simulink model "sampleModel36"  (Simulink 9.1)
settings: Solver=VariableStepAuto  StartTime=0.0  StopTime=10.0  RelTol=1e-3
undefined symbols (not defined in the file): DiscIntNeverNeededParam, Newton, Raphson
libraries: simulink x48
(part 1 of 2)
settings Model: SuppressorTable="22 serialization::archive 11 0 6 0 0 2 8 0 0 0 0 6 0 0 1 0 21 sampleModel36/cfblk78 0 6 0 0 2 8 0 0 0 0 6 41 Simulink:DataType:WarningOverFlowDetected 0 0 0 6 0  0  0 0 0 0 8 20160608 0 0 0 15 23 17 0 1 40 SimulinkFixedPoint:util:Overflowoccurred 0 0 0  0  8 20160608 0 15 23 17 0 1 1 0 21 sampleModel36/cfblk80 2 8 0 41 Simulink:DataType:WarningOverFlowDetected 0 0 0  0  8 20160523 0 10 57 55 0 1 40 SimulinkFixedPoint:util:Overflowoccurred 0 0 0  0  8 20160523 0 10 57 55 0 1"  Creator=DELL  LastModifiedBy=DELL
settings DataIOCC: SaveFormat=Dataset
settings OptimizationCC: LifeSpan=auto
settings DebuggingCC: UnderspecifiedInitializationDetection=Simplified  MergeDetectMultiDrivingBlocksExec=error  SFUnexpectedBacktrackingDiag=error  SFNoUnconditionalDefaultTransitionDiag=error  SFExecutionAtInitializationDiag=warning
settings HardwareCC: ProdBitPerPointer=64  ProdBitPerSizeT=64  ProdBitPerPtrDiffT=64  ProdLargestAtomicFloat=Float  ProdIntDivRoundTo=Zero  ProdEndianess=LittleEndian  ProdWordSize=64  ProdHWDeviceType=Intel->x86-64 (Windows64)
settings ModelReferenceCC: PropagateSignalLabelsOutOfModel=on
settings CodeAppCC: StateflowObjectComments=off
settings GRTTargetCC: TargetLangStandard=C99 (ISO)  CombineOutputUpdateFcns=on  GRTInterface=off
settings ConfigComp: CovMetricSettings=dwe  CovHtmlReporting=off  CovSaveCumulativeToWorkspaceVar=off  CovSaveSingleToWorkspaceVar=off  CovExternalEMLEnable=on

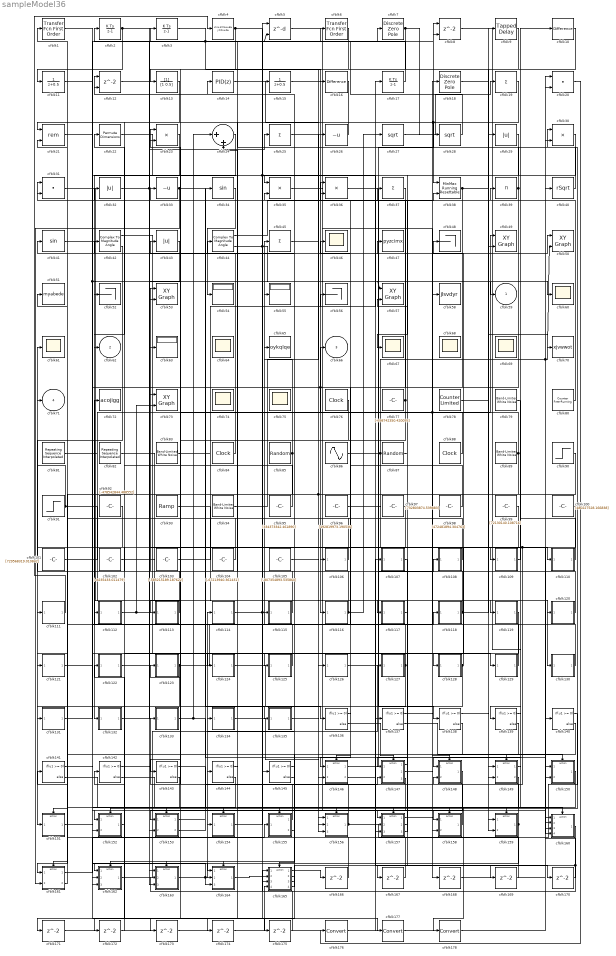
== system sampleModel36 ==
  cfblk1 : simulink/Discrete/Transfer Fcn First Order  PoleZ=0.95  ICPrevOutput=0.0  DoSatur=off
      settings: SourceProductName=Simulink
  cfblk10 : simulink/Discrete/Difference  ICPrevInput=0.0  OutMin=[]  OutMax=[]  OutDataTypeStr=Inherit: Inherit via back propagation  OutDataType=fixdt(1, 16)  OutScaling=2^-10  DoSatur=off
  cfblk100 : Constant  Value=[480227528.166838]  SampleTime=1
  cfblk101 : Constant  Value=[729568319.010842]  SampleTime=1
  cfblk102 : Constant  Value=[-8235433.011479]  SampleTime=1
  cfblk103 : Constant  Value=[-585215189.187622]  SampleTime=1
  cfblk104 : Constant  Value=[-67213940.361431]  SampleTime=1
  cfblk105 : Constant  Value=[-807354893.535860]  SampleTime=1
  cfblk106 : Subsystem
  cfblk107 : Subsystem
  cfblk108 : Subsystem
  cfblk109 : Subsystem
  cfblk11 : DiscreteTransferFcn  SampleTime=1
  cfblk110 : Subsystem
  cfblk111 : Subsystem
  cfblk112 : Subsystem
  cfblk113 : Subsystem
  cfblk114 : Subsystem
  cfblk115 : Subsystem
  cfblk116 : Subsystem
  cfblk117 : Subsystem
  cfblk118 : Subsystem
  cfblk119 : Subsystem
  cfblk12 : Delay  ShowEnablePort=on  SampleTime=1
      settings: InputPortMap=u0,e6
  cfblk120 : Subsystem
  cfblk121 : Subsystem
  cfblk122 : Subsystem
  cfblk123 : Subsystem
  cfblk124 : Subsystem
  cfblk125 : Subsystem
  cfblk126 : Subsystem
  cfblk127 : Subsystem
  cfblk128 : Subsystem
  cfblk129 : Subsystem
  cfblk13 : DiscreteFilter  SampleTime=1
  cfblk130 : Subsystem
  cfblk131 : Subsystem
  cfblk132 : Subsystem
  cfblk133 : Subsystem
  cfblk134 : Subsystem
  cfblk135 : Subsystem
  cfblk{136..145} (10 alike) : If  IfExpression=u1 >= 0  SampleTime=1
  cfblk14 : simulink/Continuous/PID Controller  Controller=PID  TimeDomain=Discrete-time  SampleTime=1  IntegratorMethod=Forward Euler  FilterMethod=Forward Euler  Form=Parallel  UseFilter=on  ControllerParametersSource=internal  P=1  I=1  D=0  N=100  InitialConditionSource=internal  InitialConditionForIntegrator=0  InitialConditionForFilter=0  ExternalReset=none  LimitOutput=off  UpperSaturationLimit=inf  LowerSaturationLimit=-inf  LinearizeAsGain=off  AntiWindupMode=none  Kb=1  TrackingMode=off  Kt=1  PParamMin=[]  PParamMax=[]  IParamMin=[]  IParamMax=[]  DParamMin=[]  DParamMax=[]  NParamMin=[]  NParamMax=[]  KbParamMin=[]  KbParamMax=[]  KtParamMin=[]  KtParamMax=[]  POutMin=[]  POutMax=[]  IOutMin=[]  IOutMax=[]  DOutMin=[]  DOutMax=[]  NOutMin=[]  NOutMax=[]  KbOutMin=[]  KbOutMax=[]  KtOutMin=[]  KtOutMax=[]  IntegratorOutMin=[]  IntegratorOutMax=[]  FilterOutMin=[]  FilterOutMax=[]  SumOutMin=[]  SumOutMax=[]  SumI1OutMin=[]  SumI1OutMax=[]  SumI2OutMin=[]  SumI2OutMax=[]  SumI3OutMin=[]  SumI3OutMax=[]  SumDOutMin=[]  SumDOutMax=[]  SaturationOutMin=[]  SaturationOutMax=[]  IntegratorContinuousStateAttributes=''  IntegratorStateMustResolveToSignalObject=off  IntegratorRTWStateStorageClass=Auto  FilterContinuousStateAttributes=''  FilterStateMustResolveToSignalObject=off  FilterRTWStateStorageClass=Auto  DifferentiatorICPrevScaledInput=0  DifferentiatorOutMin=[]  DifferentiatorOutMax=[]  FilterDiffOutCoefMin=[]  FilterDiffOutCoefMax=[]  SumDenOutMin=[]  SumDenOutMax=[]  SumNumOutMin=[]  SumNumOutMax=[]  ReciprocalOutMin=[]  ReciprocalOutMax=[]  DivideOutMin=[]  DivideOutMax=[]  TunerSelectOption=Transfer Function Based (PID Tuner App)
  cfblk146 : Subsystem  TreatAsAtomicUnit=on
  cfblk147 : Subsystem  TreatAsAtomicUnit=on
  cfblk148 : Subsystem  TreatAsAtomicUnit=on
  cfblk149 : Subsystem  TreatAsAtomicUnit=on
  cfblk15 : DiscreteTransferFcn  SampleTime=1
  cfblk150 : Subsystem  TreatAsAtomicUnit=on
  cfblk151 : Subsystem  TreatAsAtomicUnit=on
  cfblk152 : Subsystem  TreatAsAtomicUnit=on
  cfblk153 : Subsystem  TreatAsAtomicUnit=on
  cfblk154 : Subsystem  TreatAsAtomicUnit=on
  cfblk155 : Subsystem  TreatAsAtomicUnit=on
  cfblk156 : Subsystem  TreatAsAtomicUnit=on
  cfblk157 : Subsystem  TreatAsAtomicUnit=on
  cfblk158 : Subsystem  TreatAsAtomicUnit=on
  cfblk159 : Subsystem  TreatAsAtomicUnit=on
  cfblk16 : simulink/Discrete/Difference  ICPrevInput=0.0  OutMin=[]  OutMax=[]  OutDataTypeStr=Inherit: Inherit via back propagation  OutDataType=fixdt(1, 16)  OutScaling=2^-10  DoSatur=off
  cfblk160 : Subsystem  TreatAsAtomicUnit=on
  cfblk161 : Subsystem  TreatAsAtomicUnit=on
  cfblk162 : Subsystem  TreatAsAtomicUnit=on
  cfblk163 : Subsystem  TreatAsAtomicUnit=on
  cfblk164 : Subsystem  TreatAsAtomicUnit=on
  cfblk165 : Subsystem  TreatAsAtomicUnit=on
  cfblk{166..175} (10 alike) : Delay  SampleTime=1
  cfblk17 : DiscreteIntegrator  ICPrevOutput=DiscIntNeverNeededParam  ICPrevScaledInput=DiscIntNeverNeededParam
  cfblk176 : DataTypeConversion
  cfblk177 : DataTypeConversion
  cfblk178 : DataTypeConversion
  cfblk18 : DiscreteZeroPole  Poles=[0 0.5]  Gain=1
  cfblk{19,25,37,45} (4 alike) : Sum  Inputs=+
  cfblk2 : DiscreteIntegrator  ICPrevOutput=DiscIntNeverNeededParam  ICPrevScaledInput=DiscIntNeverNeededParam
  cfblk20 : DotProduct  InputSameDT=on  OutDataTypeStr=Inherit: Inherit via internal rule
  cfblk21 : Math  Operator=rem  SaturateOnIntegerOverflow=on
  cfblk22 : PermuteDimensions
  cfblk23 : Product  Inputs=**
  cfblk24 : Sum  Inputs=|++
  cfblk26 : UnaryMinus
  cfblk27 : Sqrt  SaturateOnIntegerOverflow=on
  cfblk28 : Sqrt  SaturateOnIntegerOverflow=on
  cfblk29 : Abs
  cfblk3 : DiscreteIntegrator  ICPrevOutput=DiscIntNeverNeededParam  ICPrevScaledInput=DiscIntNeverNeededParam
  cfblk30 : Product
  cfblk31 : DotProduct  InputSameDT=on  OutDataTypeStr=Inherit: Inherit via internal rule
  cfblk32 : Abs
  cfblk33 : UnaryMinus
  cfblk34 : Trigonometry
  cfblk35 : Product
  cfblk36 : Product
  cfblk38 : simulink/Math Operations/MinMax Running Resettable  Function=min  vinit=0.0
  cfblk39 : Product  Inputs=*
  cfblk4 : DiscreteStateSpace
  cfblk40 : Sqrt  Operator=rSqrt  AlgorithmType=Newton-Raphson  SaturateOnIntegerOverflow=on
  cfblk41 : Trigonometry
  cfblk42 : ComplexToMagnitudeAngle
  cfblk43 : Abs
  cfblk44 : ComplexToMagnitudeAngle
  cfblk{46,60..61,64,67..69,74..75} (9 alike) : Scope
      cfblk64 settings: Floating=on
      cfblk68 settings: Floating=on
      cfblk69 settings: Floating=on
      cfblk74 settings: Floating=on
      cfblk75 settings: Floating=on
  cfblk47 : ToWorkspace  VariableName=pyzcimx  SaveFormat=Timeseries  SampleTime=-1
  cfblk48 : Terminator
  cfblk{49..50,53,57,73} (5 alike) : simulink/Sinks/XY Graph  xmin=-1  xmax=1  ymin=-1  ymax=1  st=-1
  cfblk5 : Delay  DelayLengthSource=Input port  SampleTime=1
      settings: InputPortMap=u0,p1
  cfblk51 : ToWorkspace  VariableName=myabede  SaveFormat=Timeseries  SampleTime=-1
  cfblk52 : Terminator
  cfblk54 : Display
  cfblk55 : Display
  cfblk56 : Terminator
  cfblk58 : ToWorkspace  VariableName=jlsvdyr  SaveFormat=Timeseries  SampleTime=-1
  cfblk6 : simulink/Discrete/Transfer Fcn First Order  PoleZ=0.95  ICPrevOutput=0.0  DoSatur=off
      settings: SourceProductName=Simulink
  cfblk63 : Display
  cfblk65 : ToWorkspace  VariableName=oykqlqe  SaveFormat=Timeseries  SampleTime=-1
  cfblk7 : DiscreteZeroPole  Poles=[0 0.5]  Gain=1
  cfblk70 : ToWorkspace  VariableName=xjvwwot  SaveFormat=Timeseries  SampleTime=-1
  cfblk72 : ToWorkspace  VariableName=acojigg  SaveFormat=Timeseries  SampleTime=-1
  cfblk76 : DigitalClock
  cfblk77 : Constant  Value=[-698742350.420095]  SampleTime=1
  cfblk78 : simulink/Sources/Counter Limited  uplimit=[563.000000]  tsamp=-1
  cfblk79 : simulink/Sources/Band-Limited White Noise  Cov=[5262245646.947961]  Ts=0.1  seed=[7499573642.000000]
  cfblk8 : Delay  ShowEnablePort=on  SampleTime=1
      settings: InputPortMap=u0,e6
  cfblk80 : simulink/Sources/Counter Free-Running  NumBits=[10.000000]  tsamp=-1
  cfblk81 : simulink/Sources/Repeating Sequence Interpolated  OutValues=[-717569786.337497, -786951545.619581, 871859825.205165, -978024908.591797, -592437085.964163]  TimeValues=[0 0.1 0.5 0.6 1].'  LookUpMeth=Use Input Below  tsamp=0.01  OutMin=[]  OutMax=[]  OutDataTypeStr=double  OutputDataTypeScalingMode=double  OutDataType=fixdt(0,8)  OutScaling=2^-10
  cfblk82 : simulink/Sources/Repeating Sequence Interpolated  OutValues=[-154038240.023456, 915570522.285018, -432332103.291962, 774629816.872916, -868714883.246416]  TimeValues=[0 0.1 0.5 0.6 1].'  LookUpMeth=Use Input Above  tsamp=0.01  OutMin=[]  OutMax=[]  OutDataTypeStr=double  OutputDataTypeScalingMode=double  OutDataType=fixdt(0,8)  OutScaling=2^-10
  cfblk83 : simulink/Sources/Band-Limited White Noise  Cov=[2765316876.474610]  Ts=0.1  seed=[5715553858.000000]
  cfblk84 : DigitalClock
  cfblk85 : UniformRandomNumber  Minimum=[-3503548894.777228]  Maximum=[8747219414.346481]  Seed=[48755141.000000]  SampleTime=0.1
  cfblk86 : Sin  Amplitude=[-627808321.925341]  Bias=[-301483454.666432]  SampleTime=0
  cfblk87 : UniformRandomNumber  Minimum=[-5653446870.603408]  Maximum=[6046751050.321515]  Seed=[57719394.000000]  SampleTime=0.1
  cfblk88 : DigitalClock
  cfblk89 : simulink/Sources/Band-Limited White Noise  Cov=[5063504057.072619]  Ts=0.1  seed=[2488343886.000000]
  cfblk9 : simulink/Discrete/Tapped Delay  vinit=0.0  samptime=-1  NumDelays=1  DelayOrder=Oldest  includeCurrent=off
  cfblk90 : Step  Time=[27.000000]  Before=[545712773.558107]  After=[102090399.807930]  SampleTime=0
  cfblk91 : Step  Time=[37.000000]  Before=[895402550.988094]  After=[591374171.611668]  SampleTime=0
  cfblk92 : Constant  Value=[-478542844.488552]  SampleTime=1
  cfblk93 : simulink/Sources/Ramp  slope=[-3591.772150]  start=[40.612428]  InitialOutput=[471167.394474]
  cfblk94 : simulink/Sources/Band-Limited White Noise  Cov=[7229783405.351925]  Ts=0.1  seed=[743836585.000000]
  cfblk95 : Constant  Value=[334373342.461890]  SampleTime=1
  cfblk96 : Constant  Value=[492819973.190536]  SampleTime=1
  cfblk97 : Constant  Value=[732803874.539883]  SampleTime=1
  cfblk98 : Constant  Value=[472481894.304763]  SampleTime=1
  cfblk99 : Constant  Value=[72130140.108716]  SampleTime=1
  cfblk59 : Outport
  cfblk62 : Outport  Port=2
  cfblk66 : Outport  Port=3
  cfblk71 : Outport  Port=4
  wires:
  cfblk42/1 -> cfblk129/1(cfblk1)
  cfblk23/1 -> cfblk132/1(cfblk1)
  cfblk16/1 -> cfblk33/1
  cfblk106/1(cfblk2) -> cfblk53/1
  cfblk8/1 -> cfblk148/1(cfblk1)
  cfblk100/1 -> cfblk133/1(cfblk1), cfblk128/1(cfblk1)
  cfblk91/1 -> cfblk61/1, cfblk160/3(cfblk14)
  cfblk116/1(cfblk2) -> cfblk27/1, cfblk24/2
  cfblk163/1(cfblk2) -> cfblk114/1(cfblk1)
  cfblk109/1(cfblk2) -> cfblk10/1
  cfblk36/1 -> cfblk138/1
  cfblk17/1 -> cfblk2/1
  cfblk126/1(cfblk2) -> cfblk8/1
  cfblk5/1 -> cfblk158/1(cfblk1)
  cfblk27/1 -> cfblk19/1
  cfblk78/1 -> cfblk149/1(cfblk1)
  cfblk146/1(cfblk2) -> cfblk108/1(cfblk1)
  cfblk7/1 -> cfblk113/1(cfblk1), cfblk28/1
  cfblk124/1(cfblk2) -> cfblk136/1
  cfblk6/1 -> cfblk116/1(cfblk1)
  cfblk81/1 -> cfblk49/1
  cfblk32/1 -> cfblk110/1(cfblk1), cfblk8/2
  cfblk31/1 -> cfblk119/1(cfblk1)
  cfblk118/1(cfblk2) -> cfblk9/1, cfblk73/1
  cfblk158/1(cfblk2) -> cfblk123/1(cfblk1)
  cfblk120/1(cfblk2) -> cfblk71/1
  cfblk25/1 -> cfblk59/1
  cfblk132/1(cfblk2) -> cfblk47/1
  cfblk130/1(cfblk2) -> cfblk31/1
  cfblk39/1 -> cfblk12/1, cfblk163/3(cfblk17)
  cfblk83/1 -> cfblk17/1
  cfblk37/1 -> cfblk146/1(cfblk1)
  cfblk4/1 -> cfblk13/1, cfblk109/1(cfblk1)
  cfblk122/1(cfblk2) -> cfblk50/1
  cfblk135/1(cfblk2) -> cfblk149/2(cfblk11)
  cfblk111/1(cfblk2) -> cfblk4/1
  cfblk96/1 -> cfblk159/1(cfblk1)
  cfblk112/1(cfblk2) -> cfblk25/1, cfblk73/2
  cfblk162/1(cfblk2) -> cfblk127/1(cfblk1)
  cfblk85/1 -> cfblk143/1, cfblk65/1
  cfblk79/1 -> cfblk139/1
  cfblk99/1 -> cfblk162/1(cfblk1)
  cfblk129/1(cfblk2) -> cfblk45/1
  cfblk77/1 -> cfblk164/1(cfblk1), cfblk32/1
  cfblk12/1 -> cfblk163/1(cfblk1)
  cfblk24/1 -> cfblk52/1
  cfblk13/1 -> cfblk62/1
  cfblk103/1 -> cfblk5/1
  cfblk34/1 -> cfblk54/1
  cfblk2/1 -> cfblk11/1, cfblk160/4(cfblk15)
  cfblk87/1 -> cfblk37/1
  cfblk155/1(cfblk2) -> cfblk43/1
  cfblk115/1(cfblk2) -> cfblk55/1
  cfblk15/1 -> cfblk130/1(cfblk1)
  cfblk127/1(cfblk2) -> cfblk46/1, cfblk173/1
  cfblk108/1(cfblk2) -> cfblk63/1
  cfblk101/1 -> cfblk29/1, cfblk18/1
  cfblk43/1 -> cfblk53/2
  cfblk10/1 -> cfblk49/2
  cfblk3/1 -> cfblk16/1, cfblk5/2
  cfblk128/1(cfblk2) -> cfblk48/1, cfblk157/1(cfblk1)
  cfblk41/1 -> cfblk137/1
  cfblk97/1 -> cfblk151/1(cfblk1)
  cfblk29/1 -> cfblk67/1
  cfblk95/1 -> cfblk22/1
  cfblk110/1(cfblk2) -> cfblk39/1
  cfblk160/1(cfblk2) -> cfblk163/2(cfblk16), cfblk171/1
  cfblk94/1 -> cfblk26/1
  cfblk134/1(cfblk2) -> cfblk146/2(cfblk13)
  cfblk131/1(cfblk2) -> cfblk7/1
  cfblk28/1 -> cfblk6/1
  cfblk42/2 -> cfblk111/1(cfblk1)
  cfblk92/1 -> cfblk121/1(cfblk1)
  cfblk89/1 -> cfblk131/1(cfblk1), cfblk23/2
  cfblk156/1(cfblk2) -> cfblk30/1, cfblk23/1
  cfblk18/1 -> cfblk120/1(cfblk1)
  cfblk21/1 -> cfblk164/2(cfblk8), cfblk164/3(cfblk9), cfblk57/1
  cfblk26/1 -> cfblk21/1
  cfblk35/1 -> cfblk158/2(cfblk14)
  cfblk98/1 -> cfblk36/1
  cfblk82/1 -> cfblk150/1(cfblk1)
  cfblk107/1(cfblk2) -> cfblk147/1(cfblk1)
  cfblk161/1(cfblk2) -> cfblk155/1(cfblk1)
  cfblk113/1(cfblk2) -> cfblk42/1
  cfblk14/1 -> cfblk156/1(cfblk1)
  cfblk165/2(cfblk11) -> cfblk12/2
  cfblk152/1(cfblk2) -> cfblk122/1(cfblk1)
  cfblk104/1 -> cfblk41/1
  cfblk154/1(cfblk2) -> cfblk56/1
  cfblk161/2(cfblk10) -> cfblk51/1
  cfblk117/1(cfblk2) -> cfblk57/2
  cfblk44/1 -> cfblk36/2
  cfblk93/1 -> cfblk159/2(cfblk17)
  cfblk121/1(cfblk2) -> cfblk118/1(cfblk1)
  cfblk90/1 -> cfblk156/2(cfblk11), cfblk153/2(cfblk13)
  cfblk159/1(cfblk2) -> cfblk144/1, cfblk162/2(cfblk8)
  cfblk165/3(cfblk12) -> cfblk134/1(cfblk1)
  cfblk102/1 -> cfblk126/1(cfblk1)
  cfblk149/1(cfblk2) -> cfblk148/2(cfblk10)
  cfblk19/1 -> cfblk38/1, cfblk124/1(cfblk1)
  cfblk38/1 -> cfblk106/1(cfblk1), cfblk162/3(cfblk9), cfblk70/1
  cfblk1/1 -> cfblk35/1
  cfblk40/1 -> cfblk3/1
  cfblk133/1(cfblk2) -> cfblk150/2(cfblk13), cfblk24/1
  cfblk44/2 -> cfblk15/1, cfblk60/1
  cfblk125/1(cfblk2) -> cfblk72/1
  cfblk80/1 -> cfblk1/1
  cfblk153/1(cfblk2) -> cfblk34/1
  cfblk105/1 -> cfblk117/1(cfblk1)
  cfblk123/1(cfblk2) -> cfblk58/1, cfblk161/1(cfblk1)
  cfblk84/1 -> cfblk21/2
  cfblk45/1 -> cfblk38/2
  cfblk165/4(cfblk13) -> cfblk44/1
  cfblk157/2(cfblk14) -> cfblk112/1(cfblk1)
  cfblk86/1 -> cfblk50/2, cfblk40/1, cfblk160/2(cfblk13)
  cfblk76/1 -> cfblk153/1(cfblk1)
  cfblk22/1 -> cfblk115/1(cfblk1), cfblk145/1, cfblk157/2(cfblk12)
  cfblk11/1 -> cfblk125/1(cfblk1)
  cfblk157/3(cfblk15) -> cfblk31/2
  cfblk9/1 -> cfblk156/3(cfblk12)
  cfblk164/1(cfblk2) -> cfblk165/2(cfblk8)
  cfblk30/1 -> cfblk165/3(cfblk9)
  cfblk88/1 -> cfblk66/1
  cfblk33/1 -> cfblk135/1(cfblk1), cfblk161/2(cfblk9)
  cfblk155/2(cfblk13) -> cfblk14/1
  cfblk153/2(cfblk14) -> cfblk147/2(cfblk14)
  cfblk148/1(cfblk2) -> cfblk152/1(cfblk1)
  cfblk147/3(cfblk16) -> cfblk152/2(cfblk8)
  cfblk136/1 -> cfblk146/Action
  cfblk136/2 -> cfblk147/Action
  cfblk137/1 -> cfblk148/Action
  cfblk137/2 -> cfblk149/Action
  cfblk138/1 -> cfblk150/Action
  cfblk138/2 -> cfblk151/Action
  cfblk139/1 -> cfblk152/Action
  cfblk139/2 -> cfblk153/Action
  cfblk140/1 -> cfblk154/Action
  cfblk140/2 -> cfblk155/Action
  cfblk141/1 -> cfblk156/Action
  cfblk141/2 -> cfblk157/Action
  cfblk142/1 -> cfblk158/Action
  cfblk142/2 -> cfblk159/Action
  cfblk143/1 -> cfblk160/Action
  cfblk143/2 -> cfblk161/Action
  cfblk144/1 -> cfblk162/Action
  cfblk144/2 -> cfblk163/Action
  cfblk145/1 -> cfblk164/Action
  cfblk145/2 -> cfblk165/Action
  cfblk165/1(cfblk2) -> cfblk166/1
  cfblk166/1 -> cfblk154/1(cfblk1)
  cfblk147/1(cfblk2) -> cfblk167/1
  cfblk167/1 -> cfblk35/2
  cfblk147/2(cfblk15) -> cfblk168/1
  cfblk168/1 -> cfblk30/2
  cfblk146/2(cfblk14) -> cfblk169/1
  cfblk169/1 -> cfblk141/1
  cfblk157/1(cfblk2) -> cfblk170/1
  cfblk170/1 -> cfblk160/1(cfblk1)
  cfblk171/1 -> cfblk157/3(cfblk13)
  cfblk119/1(cfblk2) -> cfblk172/1
  cfblk172/1 -> cfblk142/1
  cfblk173/1 -> cfblk165/4(cfblk10)
  cfblk150/1(cfblk2) -> cfblk174/1
  cfblk174/1 -> cfblk140/1
  cfblk151/1(cfblk2) -> cfblk175/1
  cfblk175/1 -> cfblk165/1(cfblk1)
  cfblk20/1 -> cfblk176/1
  cfblk176/1 -> cfblk107/1(cfblk1)
  cfblk114/1(cfblk2) -> cfblk177/1
  cfblk177/1 -> cfblk20/1
  cfblk149/2(cfblk12) -> cfblk178/1
  cfblk178/1 -> cfblk20/2

== system sampleModel36/cfblk106 ==
  cfblk1 : Inport
  cfblk2 : Outport
  wires:
  cfblk1/1 -> cfblk2/1

== system sampleModel36/cfblk107 ==
  cfblk1 : Inport
  cfblk2 : Outport
  wires:
  cfblk1/1 -> cfblk2/1

== system sampleModel36/cfblk108 ==
  cfblk1 : Inport
  cfblk2 : Outport
  wires:
  cfblk1/1 -> cfblk2/1

== system sampleModel36/cfblk109 ==
  cfblk1 : Inport
  cfblk2 : Outport
  wires:
  cfblk1/1 -> cfblk2/1

== system sampleModel36/cfblk110 ==
  cfblk1 : Inport
  cfblk2 : Outport
  wires:
  cfblk1/1 -> cfblk2/1

== system sampleModel36/cfblk111 ==
  cfblk1 : Inport
  cfblk2 : Outport
  wires:
  cfblk1/1 -> cfblk2/1

== system sampleModel36/cfblk112 ==
  cfblk1 : Inport
  cfblk2 : Outport
  wires:
  cfblk1/1 -> cfblk2/1

== system sampleModel36/cfblk113 ==
  cfblk1 : Inport
  cfblk2 : Outport
  wires:
  cfblk1/1 -> cfblk2/1

== system sampleModel36/cfblk114 ==
  cfblk1 : Inport
  cfblk2 : Outport
  wires:
  cfblk1/1 -> cfblk2/1

== system sampleModel36/cfblk115 ==
  cfblk1 : Inport
  cfblk2 : Outport
  wires:
  cfblk1/1 -> cfblk2/1

== system sampleModel36/cfblk116 ==
  cfblk1 : Inport
  cfblk2 : Outport
  wires:
  cfblk1/1 -> cfblk2/1

== system sampleModel36/cfblk117 ==
  cfblk1 : Inport
  cfblk2 : Outport
  wires:
  cfblk1/1 -> cfblk2/1

== system sampleModel36/cfblk118 ==
  cfblk1 : Inport
  cfblk2 : Outport
  wires:
  cfblk1/1 -> cfblk2/1

== system sampleModel36/cfblk119 ==
  cfblk1 : Inport
  cfblk2 : Outport
  wires:
  cfblk1/1 -> cfblk2/1

== system sampleModel36/cfblk120 ==
  cfblk1 : Inport
  cfblk2 : Outport
  wires:
  cfblk1/1 -> cfblk2/1

== system sampleModel36/cfblk121 ==
  cfblk1 : Inport
  cfblk2 : Outport
  wires:
  cfblk1/1 -> cfblk2/1

== system sampleModel36/cfblk122 ==
  cfblk1 : Inport
  cfblk2 : Outport
  wires:
  cfblk1/1 -> cfblk2/1

== system sampleModel36/cfblk123 ==
  cfblk1 : Inport
  cfblk2 : Outport
  wires:
  cfblk1/1 -> cfblk2/1

== system sampleModel36/cfblk124 ==
  cfblk1 : Inport
  cfblk2 : Outport
  wires:
  cfblk1/1 -> cfblk2/1

== system sampleModel36/cfblk125 ==
  cfblk1 : Inport
  cfblk2 : Outport
  wires:
  cfblk1/1 -> cfblk2/1

== system sampleModel36/cfblk126 ==
  cfblk1 : Inport
  cfblk2 : Outport
  wires:
  cfblk1/1 -> cfblk2/1

== system sampleModel36/cfblk127 ==
  cfblk1 : Inport
  cfblk2 : Outport
  wires:
  cfblk1/1 -> cfblk2/1

== system sampleModel36/cfblk128 ==
  cfblk1 : Inport
  cfblk2 : Outport
  wires:
  cfblk1/1 -> cfblk2/1

== system sampleModel36/cfblk129 ==
  cfblk1 : Inport
  cfblk2 : Outport
  wires:
  cfblk1/1 -> cfblk2/1

== system sampleModel36/cfblk130 ==
  cfblk1 : Inport
  cfblk2 : Outport
  wires:
  cfblk1/1 -> cfblk2/1

== system sampleModel36/cfblk131 ==
  cfblk1 : Inport
  cfblk2 : Outport
  wires:
  cfblk1/1 -> cfblk2/1

== system sampleModel36/cfblk132 ==
  cfblk1 : Inport
  cfblk2 : Outport
  wires:
  cfblk1/1 -> cfblk2/1

== system sampleModel36/cfblk133 ==
  cfblk1 : Inport
  cfblk2 : Outport
  wires:
  cfblk1/1 -> cfblk2/1

== system sampleModel36/cfblk134 ==
  cfblk1 : Inport
  cfblk2 : Outport
  wires:
  cfblk1/1 -> cfblk2/1

== system sampleModel36/cfblk135 ==
  cfblk1 : Inport
  cfblk2 : Outport
  wires:
  cfblk1/1 -> cfblk2/1

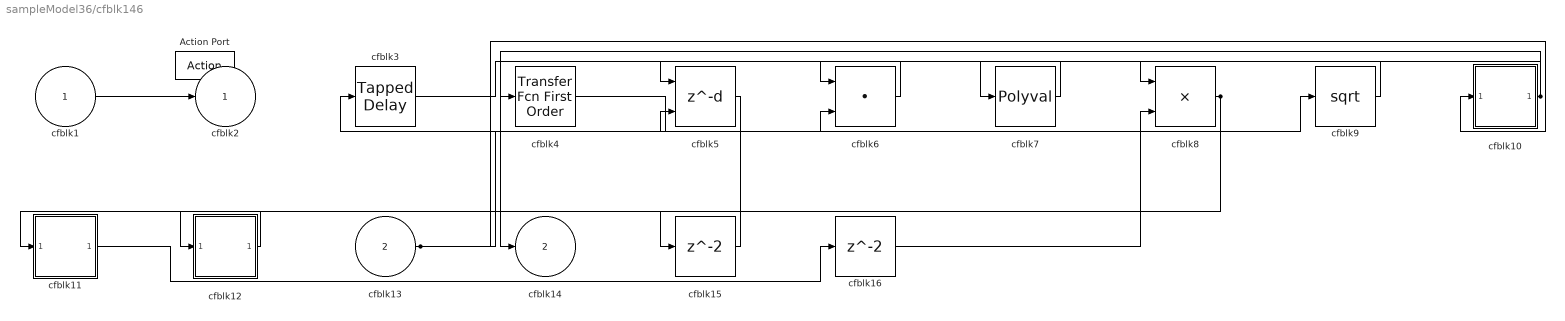
== system sampleModel36/cfblk146 ==
  cfblk1 : Inport
  cfblk13 : Inport  Port=2
  Action Port : ActionPort  ActionType=then
  cfblk10 : Subsystem
  cfblk11 : Subsystem
  cfblk12 : Subsystem
  cfblk15 : Delay
  cfblk16 : Delay
  cfblk3 : simulink/Discrete/Tapped Delay  vinit=0.0  samptime=-1  NumDelays=1  DelayOrder=Oldest  includeCurrent=off
  cfblk4 : simulink/Discrete/Transfer Fcn First Order  PoleZ=0.95  ICPrevOutput=0.0  DoSatur=off
      settings: SourceProductName=Simulink
  cfblk5 : Delay  DelayLengthSource=Input port
      settings: InputPortMap=u0,p1
  cfblk6 : DotProduct  InputSameDT=on  OutDataTypeStr=Inherit: Inherit via internal rule
  cfblk7 : Polyval  Coefs=[ +2.081618890e-019, -1.441693666e-014, +4.719686976e-010, -8.536869453e-006, +1.621573104e-001, -8.087801117e+001 ]
  cfblk8 : Product  Inputs=**
  cfblk9 : Sqrt  SaturateOnIntegerOverflow=on
  cfblk2 : Outport
  cfblk14 : Outport  Port=2
  wires:
  cfblk12/1(cfblk2) -> cfblk11/1(cfblk1)
  cfblk9/1 -> cfblk8/1
  cfblk10/1(cfblk2) -> cfblk14/1, cfblk7/1
  cfblk13/1 -> cfblk10/1(cfblk1), cfblk5/2
  cfblk6/1 -> cfblk5/1
  cfblk7/1 -> cfblk4/1
  cfblk4/1 -> cfblk9/1
  cfblk1/1 -> cfblk2/1
  cfblk3/1 -> cfblk6/1
  cfblk8/1 -> cfblk12/1(cfblk1), cfblk6/2
  cfblk5/1 -> cfblk15/1
  cfblk15/1 -> cfblk3/1
  cfblk11/1(cfblk2) -> cfblk16/1
  cfblk16/1 -> cfblk8/2

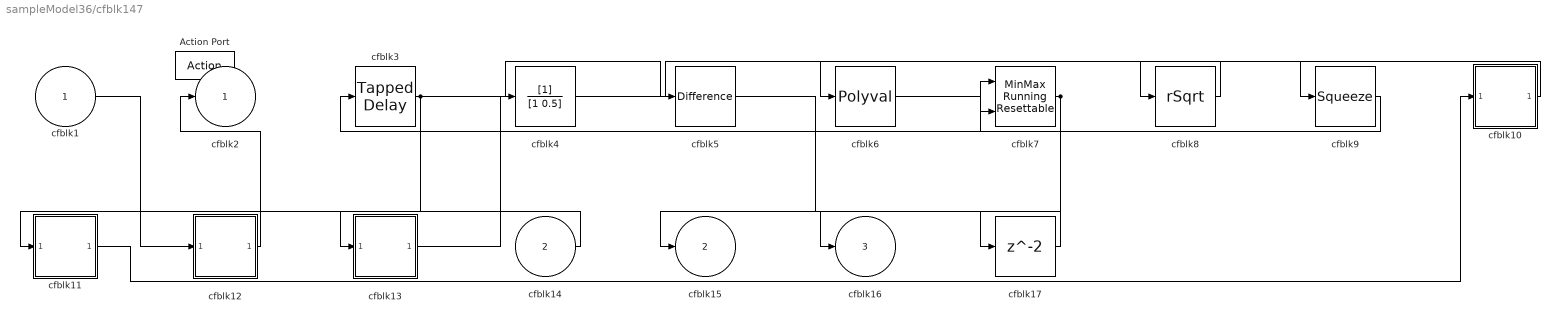
== system sampleModel36/cfblk147 ==
  cfblk1 : Inport
  cfblk14 : Inport  Port=2
  Action Port : ActionPort  ActionType=else
  cfblk10 : Subsystem
  cfblk11 : Subsystem
  cfblk12 : Subsystem
  cfblk13 : Subsystem
  cfblk17 : Delay
  cfblk3 : simulink/Discrete/Tapped Delay  vinit=0.0  samptime=-1  NumDelays=1  DelayOrder=Oldest  includeCurrent=off
  cfblk4 : DiscreteFilter
  cfblk5 : simulink/Discrete/Difference  ICPrevInput=0.0  OutMin=[]  OutMax=[]  OutDataTypeStr=Inherit: Inherit via back propagation  OutDataType=fixdt(1, 16)  OutScaling=2^-10  DoSatur=off
  cfblk6 : Polyval  Coefs=[ +2.081618890e-019, -1.441693666e-014, +4.719686976e-010, -8.536869453e-006, +1.621573104e-001, -8.087801117e+001 ]
  cfblk7 : simulink/Math Operations/MinMax Running Resettable  Function=min  vinit=0.0
  cfblk8 : Sqrt  Operator=rSqrt  AlgorithmType=Newton-Raphson  SaturateOnIntegerOverflow=on
  cfblk9 : Squeeze
  cfblk2 : Outport
  cfblk15 : Outport  Port=2
  cfblk16 : Outport  Port=3
  wires:
  cfblk4/1 -> cfblk9/1
  cfblk9/1 -> cfblk7/1
  cfblk8/1 -> cfblk6/1
  cfblk12/1(cfblk2) -> cfblk2/1
  cfblk3/1 -> cfblk5/1, cfblk11/1(cfblk1)
  cfblk10/1(cfblk2) -> cfblk8/1
  cfblk6/1 -> cfblk7/2
  cfblk1/1 -> cfblk12/1(cfblk1)
  cfblk14/1 -> cfblk13/1(cfblk1)
  cfblk7/1 -> cfblk16/1, cfblk15/1
  cfblk13/1(cfblk2) -> cfblk4/1
  cfblk11/1(cfblk2) -> cfblk10/1(cfblk1)
  cfblk5/1 -> cfblk17/1
  cfblk17/1 -> cfblk3/1

== system sampleModel36/cfblk148 ==
  cfblk1 : Inport
  cfblk10 : Inport  Port=2
  Action Port : ActionPort  ActionType=then
  cfblk3 : Product  Inputs=**
  cfblk4 : DotProduct  InputSameDT=on  OutDataTypeStr=Inherit: Inherit via internal rule
  cfblk5 : Product
  cfblk6 : Sqrt  SaturateOnIntegerOverflow=on
  cfblk7 : Constant  Value=[530901594.292365]  SampleTime=1
  cfblk8 : Subsystem
  cfblk9 : Subsystem
  cfblk2 : Outport
  wires:
  cfblk5/1 -> cfblk8/1(cfblk1)
  cfblk10/1 -> cfblk9/1(cfblk1)
  cfblk8/1(cfblk2) -> cfblk4/1
  cfblk3/1 -> cfblk6/1
  cfblk6/1 -> cfblk4/2
  cfblk7/1 -> cfblk5/1, cfblk5/2
  cfblk4/1 -> cfblk2/1
  cfblk9/1(cfblk2) -> cfblk3/1
  cfblk1/1 -> cfblk3/2

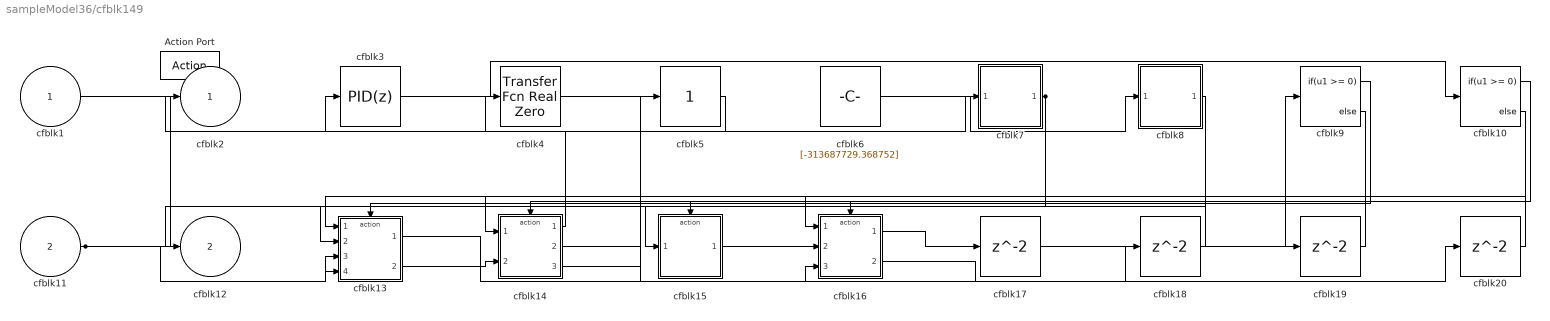
== system sampleModel36/cfblk149 ==
  cfblk1 : Inport
  cfblk11 : Inport  Port=2
  Action Port : ActionPort  ActionType=else
  cfblk10 : If  IfExpression=u1 >= 0  SampleTime=1
  cfblk13 : Subsystem  TreatAsAtomicUnit=on
  cfblk14 : Subsystem  TreatAsAtomicUnit=on
  cfblk15 : Subsystem  TreatAsAtomicUnit=on
  cfblk16 : Subsystem  TreatAsAtomicUnit=on
  cfblk{17..20} (4 alike) : Delay
  cfblk3 : simulink/Continuous/PID Controller  Controller=PID  TimeDomain=Discrete-time  SampleTime=-1  IntegratorMethod=Forward Euler  FilterMethod=Forward Euler  Form=Parallel  UseFilter=on  ControllerParametersSource=internal  P=1  I=1  D=0  N=100  InitialConditionSource=internal  InitialConditionForIntegrator=0  InitialConditionForFilter=0  ExternalReset=none  LimitOutput=off  UpperSaturationLimit=inf  LowerSaturationLimit=-inf  LinearizeAsGain=off  AntiWindupMode=none  Kb=1  TrackingMode=off  Kt=1  PParamMin=[]  PParamMax=[]  IParamMin=[]  IParamMax=[]  DParamMin=[]  DParamMax=[]  NParamMin=[]  NParamMax=[]  KbParamMin=[]  KbParamMax=[]  KtParamMin=[]  KtParamMax=[]  POutMin=[]  POutMax=[]  IOutMin=[]  IOutMax=[]  DOutMin=[]  DOutMax=[]  NOutMin=[]  NOutMax=[]  KbOutMin=[]  KbOutMax=[]  KtOutMin=[]  KtOutMax=[]  IntegratorOutMin=[]  IntegratorOutMax=[]  FilterOutMin=[]  FilterOutMax=[]  SumOutMin=[]  SumOutMax=[]  SumI1OutMin=[]  SumI1OutMax=[]  SumI2OutMin=[]  SumI2OutMax=[]  SumI3OutMin=[]  SumI3OutMax=[]  SumDOutMin=[]  SumDOutMax=[]  SaturationOutMin=[]  SaturationOutMax=[]  IntegratorContinuousStateAttributes=''  IntegratorStateMustResolveToSignalObject=off  IntegratorRTWStateStorageClass=Auto  FilterContinuousStateAttributes=''  FilterStateMustResolveToSignalObject=off  FilterRTWStateStorageClass=Auto  DifferentiatorICPrevScaledInput=0  DifferentiatorOutMin=[]  DifferentiatorOutMax=[]  FilterDiffOutCoefMin=[]  FilterDiffOutCoefMax=[]  SumDenOutMin=[]  SumDenOutMax=[]  SumNumOutMin=[]  SumNumOutMax=[]  ReciprocalOutMin=[]  ReciprocalOutMax=[]  DivideOutMin=[]  DivideOutMax=[]  TunerSelectOption=Transfer Function Based (PID Tuner App)
  cfblk4 : simulink/Discrete/Transfer Fcn Real Zero  ZeroZ=0.75  ICPrevInput=0.0  DoSatur=off
      settings: SourceProductName=Simulink  SourceProductBaseCode=SL
  cfblk5 : simulink/Math Operations/Slider Gain  gain=1  low=0  high=2
  cfblk6 : Constant  Value=[-313687729.368752]  SampleTime=1
  cfblk7 : Subsystem
  cfblk8 : Subsystem
  cfblk9 : If  IfExpression=u1 >= 0  SampleTime=1
  cfblk2 : Outport
  cfblk12 : Outport  Port=2
  wires:
  cfblk11/1 -> cfblk3/1, cfblk13/3(cfblk11), cfblk13/4(cfblk12)
  cfblk3/1 -> cfblk10/1
  cfblk5/1 -> cfblk4/1
  cfblk6/1 -> cfblk8/1(cfblk1)
  cfblk1/1 -> cfblk7/1(cfblk1)
  cfblk8/1(cfblk2) -> cfblk15/1(cfblk1)
  cfblk7/1(cfblk2) -> cfblk12/1, cfblk13/2(cfblk10)
  cfblk14/1(cfblk2) -> cfblk2/1
  cfblk15/1(cfblk2) -> cfblk16/2(cfblk10)
  cfblk13/1(cfblk2) -> cfblk16/3(cfblk11)
  cfblk14/3(cfblk15) -> cfblk5/1
  cfblk13/2(cfblk13) -> cfblk14/2(cfblk13)
  cfblk9/1 -> cfblk13/Action
  cfblk9/2 -> cfblk14/Action
  cfblk10/1 -> cfblk15/Action
  cfblk10/2 -> cfblk16/Action
  cfblk16/1(cfblk2) -> cfblk17/1
  cfblk17/1 -> cfblk9/1
  cfblk14/2(cfblk14) -> cfblk18/1
  cfblk18/1 -> cfblk16/1(cfblk1)
  cfblk4/1 -> cfblk19/1
  cfblk19/1 -> cfblk13/1(cfblk1)
  cfblk16/2(cfblk12) -> cfblk20/1
  cfblk20/1 -> cfblk14/1(cfblk1)

== system sampleModel36/cfblk150 ==
  cfblk1 : Inport
  cfblk13 : Inport  Port=2
  Action Port : ActionPort  ActionType=then
  cfblk10 : Subsystem
  cfblk11 : Subsystem
  cfblk12 : Subsystem
  cfblk14 : Delay
  cfblk3 : simulink/Continuous/PID Controller  Controller=PID  TimeDomain=Discrete-time  SampleTime=-1  IntegratorMethod=Forward Euler  FilterMethod=Forward Euler  Form=Parallel  UseFilter=on  ControllerParametersSource=internal  P=1  I=1  D=0  N=100  InitialConditionSource=internal  InitialConditionForIntegrator=0  InitialConditionForFilter=0  ExternalReset=none  LimitOutput=off  UpperSaturationLimit=inf  LowerSaturationLimit=-inf  LinearizeAsGain=off  AntiWindupMode=none  Kb=1  TrackingMode=off  Kt=1  PParamMin=[]  PParamMax=[]  IParamMin=[]  IParamMax=[]  DParamMin=[]  DParamMax=[]  NParamMin=[]  NParamMax=[]  KbParamMin=[]  KbParamMax=[]  KtParamMin=[]  KtParamMax=[]  POutMin=[]  POutMax=[]  IOutMin=[]  IOutMax=[]  DOutMin=[]  DOutMax=[]  NOutMin=[]  NOutMax=[]  KbOutMin=[]  KbOutMax=[]  KtOutMin=[]  KtOutMax=[]  IntegratorOutMin=[]  IntegratorOutMax=[]  FilterOutMin=[]  FilterOutMax=[]  SumOutMin=[]  SumOutMax=[]  SumI1OutMin=[]  SumI1OutMax=[]  SumI2OutMin=[]  SumI2OutMax=[]  SumI3OutMin=[]  SumI3OutMax=[]  SumDOutMin=[]  SumDOutMax=[]  SaturationOutMin=[]  SaturationOutMax=[]  IntegratorContinuousStateAttributes=''  IntegratorStateMustResolveToSignalObject=off  IntegratorRTWStateStorageClass=Auto  FilterContinuousStateAttributes=''  FilterStateMustResolveToSignalObject=off  FilterRTWStateStorageClass=Auto  DifferentiatorICPrevScaledInput=0  DifferentiatorOutMin=[]  DifferentiatorOutMax=[]  FilterDiffOutCoefMin=[]  FilterDiffOutCoefMax=[]  SumDenOutMin=[]  SumDenOutMax=[]  SumNumOutMin=[]  SumNumOutMax=[]  ReciprocalOutMin=[]  ReciprocalOutMax=[]  DivideOutMin=[]  DivideOutMax=[]  TunerSelectOption=Transfer Function Based (PID Tuner App)
  cfblk4 : ComplexToRealImag
  cfblk5 : Sqrt  SaturateOnIntegerOverflow=on
  cfblk6 : Constant  Value=[305171337.768058]  SampleTime=1
  cfblk7 : Subsystem
  cfblk8 : Subsystem
  cfblk9 : Subsystem
  cfblk2 : Outport
  wires:
  cfblk8/1(cfblk2) -> cfblk11/1(cfblk1)
  cfblk4/1 -> cfblk7/1(cfblk1)
  cfblk1/1 -> cfblk12/1(cfblk1)
  cfblk13/1 -> cfblk3/1
  cfblk4/2 -> cfblk9/1(cfblk1)
  cfblk12/1(cfblk2) -> cfblk10/1(cfblk1)
  cfblk5/1 -> cfblk2/1
  cfblk11/1(cfblk2) -> cfblk5/1
  cfblk3/1 -> cfblk8/1(cfblk1)
  cfblk7/1(cfblk2) -> cfblk14/1
  cfblk14/1 -> cfblk4/1

== system sampleModel36/cfblk151 ==
  cfblk1 : Inport
  Action Port : ActionPort  ActionType=else
  cfblk10 : Constant  Value=[779105672.515790]  SampleTime=1
  cfblk11 : Delay
  cfblk3 : DiscreteFilter
  cfblk4 : DiscreteIntegrator  SampleTime=-1  ICPrevOutput=DiscIntNeverNeededParam  ICPrevScaledInput=DiscIntNeverNeededParam
  cfblk5 : simulink/Discrete/Transfer Fcn First Order  PoleZ=0.95  ICPrevOutput=0.0  DoSatur=off
      settings: SourceProductName=Simulink
  cfblk6 : DiscreteFilter
  cfblk7 : Sqrt  SaturateOnIntegerOverflow=on
  cfblk8 : Sum  Inputs=|++
  cfblk9 : Trigonometry
  cfblk2 : Outport
  wires:
  cfblk3/1 -> cfblk2/1
  cfblk1/1 -> cfblk5/1
  cfblk4/1 -> cfblk6/1
  cfblk9/1 -> cfblk8/1
  cfblk6/1 -> cfblk7/1
  cfblk5/1 -> cfblk8/2
  cfblk8/1 -> cfblk3/1
  cfblk10/1 -> cfblk9/1
  cfblk7/1 -> cfblk11/1
  cfblk11/1 -> cfblk4/1

== system sampleModel36/cfblk152 ==
  cfblk1 : Inport
  cfblk8 : Inport  Port=2
  Action Port : ActionPort  ActionType=then
  cfblk3 : simulink/Continuous/PID Controller  Controller=PID  TimeDomain=Discrete-time  SampleTime=-1  IntegratorMethod=Forward Euler  FilterMethod=Forward Euler  Form=Parallel  UseFilter=on  ControllerParametersSource=internal  P=1  I=1  D=0  N=100  InitialConditionSource=internal  InitialConditionForIntegrator=0  InitialConditionForFilter=0  ExternalReset=none  LimitOutput=off  UpperSaturationLimit=inf  LowerSaturationLimit=-inf  LinearizeAsGain=off  AntiWindupMode=none  Kb=1  TrackingMode=off  Kt=1  PParamMin=[]  PParamMax=[]  IParamMin=[]  IParamMax=[]  DParamMin=[]  DParamMax=[]  NParamMin=[]  NParamMax=[]  KbParamMin=[]  KbParamMax=[]  KtParamMin=[]  KtParamMax=[]  POutMin=[]  POutMax=[]  IOutMin=[]  IOutMax=[]  DOutMin=[]  DOutMax=[]  NOutMin=[]  NOutMax=[]  KbOutMin=[]  KbOutMax=[]  KtOutMin=[]  KtOutMax=[]  IntegratorOutMin=[]  IntegratorOutMax=[]  FilterOutMin=[]  FilterOutMax=[]  SumOutMin=[]  SumOutMax=[]  SumI1OutMin=[]  SumI1OutMax=[]  SumI2OutMin=[]  SumI2OutMax=[]  SumI3OutMin=[]  SumI3OutMax=[]  SumDOutMin=[]  SumDOutMax=[]  SaturationOutMin=[]  SaturationOutMax=[]  IntegratorContinuousStateAttributes=''  IntegratorStateMustResolveToSignalObject=off  IntegratorRTWStateStorageClass=Auto  FilterContinuousStateAttributes=''  FilterStateMustResolveToSignalObject=off  FilterRTWStateStorageClass=Auto  DifferentiatorICPrevScaledInput=0  DifferentiatorOutMin=[]  DifferentiatorOutMax=[]  FilterDiffOutCoefMin=[]  FilterDiffOutCoefMax=[]  SumDenOutMin=[]  SumDenOutMax=[]  SumNumOutMin=[]  SumNumOutMax=[]  ReciprocalOutMin=[]  ReciprocalOutMax=[]  DivideOutMin=[]  DivideOutMax=[]  TunerSelectOption=Transfer Function Based (PID Tuner App)
  cfblk4 : Product  Inputs=*
  cfblk5 : Constant  Value=[892384230.710558]  SampleTime=1
  cfblk6 : Subsystem
  cfblk7 : Subsystem
  cfblk2 : Outport
  wires:
  cfblk1/1 -> cfblk3/1
  cfblk5/1 -> cfblk2/1
  cfblk8/1 -> cfblk7/1(cfblk1)
  cfblk7/1(cfblk2) -> cfblk6/1(cfblk1)
  cfblk6/1(cfblk2) -> cfblk4/1

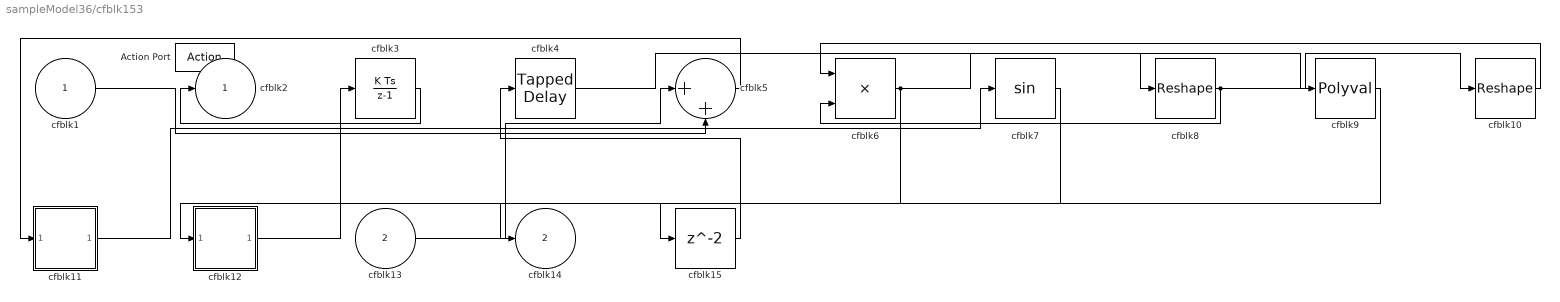
== system sampleModel36/cfblk153 ==
  cfblk1 : Inport
  cfblk13 : Inport  Port=2
  Action Port : ActionPort  ActionType=else
  cfblk10 : Reshape
  cfblk11 : Subsystem
  cfblk12 : Subsystem
  cfblk15 : Delay
  cfblk3 : DiscreteIntegrator  SampleTime=-1  ICPrevOutput=DiscIntNeverNeededParam  ICPrevScaledInput=DiscIntNeverNeededParam
  cfblk4 : simulink/Discrete/Tapped Delay  vinit=0.0  samptime=-1  NumDelays=1  DelayOrder=Oldest  includeCurrent=off
  cfblk5 : Sum  Inputs=|++
  cfblk6 : Product
  cfblk7 : Trigonometry
  cfblk8 : Reshape
  cfblk9 : Polyval  Coefs=[ +2.081618890e-019, -1.441693666e-014, +4.719686976e-010, -8.536869453e-006, +1.621573104e-001, -8.087801117e+001 ]
  cfblk2 : Outport
  cfblk14 : Outport  Port=2
  wires:
  cfblk9/1 -> cfblk12/1(cfblk1)
  cfblk11/1(cfblk2) -> cfblk7/1
  cfblk3/1 -> cfblk2/1
  cfblk8/1 -> cfblk10/1, cfblk6/2
  cfblk5/1 -> cfblk11/1(cfblk1)
  cfblk10/1 -> cfblk6/1
  cfblk12/1(cfblk2) -> cfblk3/1
  cfblk6/1 -> cfblk9/1, cfblk15/1
  cfblk13/1 -> cfblk5/1
  cfblk1/1 -> cfblk5/2
  cfblk4/1 -> cfblk8/1
  cfblk7/1 -> cfblk14/1
  cfblk15/1 -> cfblk4/1

== system sampleModel36/cfblk154 ==
  cfblk1 : Inport
  Action Port : ActionPort  ActionType=then
  cfblk3 : simulink/Discrete/Transfer Fcn Real Zero  ZeroZ=0.75  ICPrevInput=0.0  DoSatur=off
      settings: SourceProductName=Simulink  SourceProductBaseCode=SL
  cfblk4 : Delay  ShowEnablePort=on
      settings: InputPortMap=u0,e6
  cfblk5 : Sum  Inputs=|++
  cfblk6 : Math  Operator=transpose  SaturateOnIntegerOverflow=on
  cfblk7 : Squeeze
  cfblk8 : Constant  Value=[-660892011.357269]  SampleTime=1
  cfblk9 : Subsystem
  cfblk2 : Outport
  wires:
  cfblk9/1(cfblk2) -> cfblk3/1
  cfblk6/1 -> cfblk7/1
  cfblk3/1 -> cfblk5/1
  cfblk1/1 -> cfblk6/1
  cfblk7/1 -> cfblk4/1, cfblk9/1(cfblk1)
  cfblk4/1 -> cfblk2/1
  cfblk8/1 -> cfblk5/2
  cfblk5/1 -> cfblk4/2

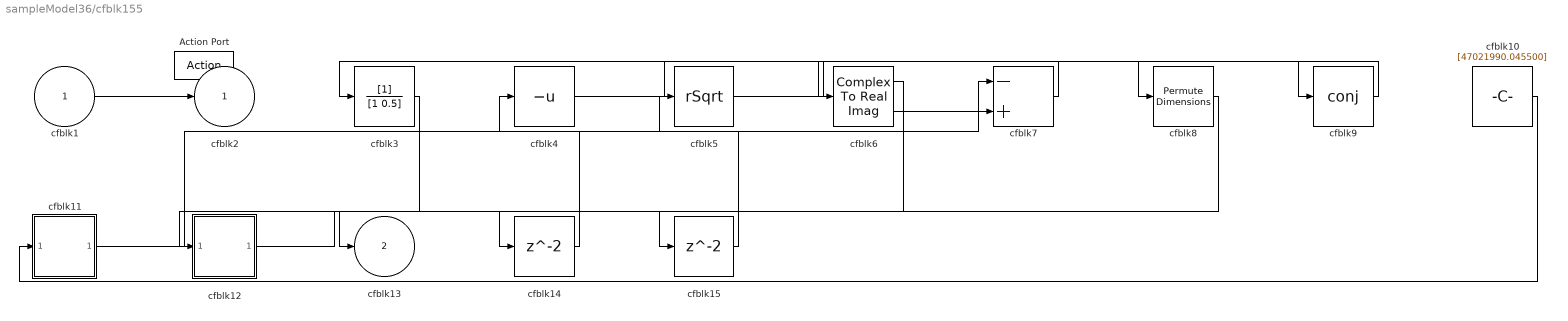
== system sampleModel36/cfblk155 ==
  cfblk1 : Inport
  Action Port : ActionPort  ActionType=else
  cfblk10 : Constant  Value=[47021990.045500]  SampleTime=1
  cfblk11 : Subsystem
  cfblk12 : Subsystem
  cfblk14 : Delay
  cfblk15 : Delay
  cfblk3 : DiscreteFilter
  cfblk4 : UnaryMinus
  cfblk5 : Sqrt  Operator=rSqrt  AlgorithmType=Newton-Raphson  SaturateOnIntegerOverflow=on
  cfblk6 : ComplexToRealImag
  cfblk7 : Sum  Inputs=-+
  cfblk8 : PermuteDimensions
  cfblk9 : Math  Operator=conj  SaturateOnIntegerOverflow=on
  cfblk2 : Outport
  cfblk13 : Outport  Port=2
  wires:
  cfblk4/1 -> cfblk8/1
  cfblk11/1(cfblk2) -> cfblk7/1
  cfblk6/1 -> cfblk12/1(cfblk1)
  cfblk7/1 -> cfblk3/1
  cfblk5/1 -> cfblk9/1
  cfblk9/1 -> cfblk6/1
  cfblk6/2 -> cfblk7/2
  cfblk10/1 -> cfblk11/1(cfblk1)
  cfblk3/1 -> cfblk13/1
  cfblk1/1 -> cfblk2/1
  cfblk8/1 -> cfblk14/1
  cfblk14/1 -> cfblk4/1
  cfblk12/1(cfblk2) -> cfblk15/1
  cfblk15/1 -> cfblk5/1

== system sampleModel36/cfblk156 ==
  cfblk1 : Inport
  cfblk11 : Inport  Port=2
  cfblk12 : Inport  Port=3
  Action Port : ActionPort  ActionType=then
  cfblk10 : Subsystem
  cfblk3 : Delay
  cfblk4 : Delay  ShowEnablePort=on
      settings: InputPortMap=u0,e6
  cfblk5 : Reshape
  cfblk6 : Sqrt  Operator=rSqrt  AlgorithmType=Newton-Raphson  SaturateOnIntegerOverflow=on
  cfblk7 : Constant  Value=[-521772301.207292]  SampleTime=1
  cfblk8 : Subsystem
  cfblk9 : Subsystem
  cfblk2 : Outport
  wires:
  cfblk11/1 -> cfblk3/1
  cfblk6/1 -> cfblk5/1
  cfblk7/1 -> cfblk2/1
  cfblk5/1 -> cfblk4/1
  cfblk3/1 -> cfblk4/2
  cfblk10/1(cfblk2) -> cfblk8/1(cfblk1)
  cfblk12/1 -> cfblk9/1(cfblk1)
  cfblk9/1(cfblk2) -> cfblk10/1(cfblk1)
  cfblk1/1 -> cfblk6/1

== system sampleModel36/cfblk157 ==
  cfblk1 : Inport
  cfblk12 : Inport  Port=2
  cfblk13 : Inport  Port=3
  Action Port : ActionPort  ActionType=else
  cfblk10 : Subsystem
  cfblk11 : Subsystem
  cfblk3 : DiscreteFir
  cfblk4 : simulink/Discrete/Difference  ICPrevInput=0.0  OutMin=[]  OutMax=[]  OutDataTypeStr=Inherit: Inherit via back propagation  OutDataType=fixdt(1, 16)  OutScaling=2^-10  DoSatur=off
  cfblk5 : Rounding
  cfblk6 : Constant  Value=[-604714890.223257]  SampleTime=1
  cfblk7 : Constant  Value=[306518758.648467]  SampleTime=1
  cfblk8 : Constant  Value=[430265041.779054]  SampleTime=1
  cfblk9 : Subsystem
  cfblk2 : Outport
  cfblk14 : Outport  Port=2
  cfblk15 : Outport  Port=3
  wires:
  cfblk8/1 -> cfblk4/1
  cfblk1/1 -> cfblk15/1
  cfblk5/1 -> cfblk3/1
  cfblk12/1 -> cfblk5/1
  cfblk4/1 -> cfblk9/1(cfblk1)
  cfblk7/1 -> cfblk2/1
  cfblk6/1 -> cfblk11/1(cfblk1)
  cfblk9/1(cfblk2) -> cfblk10/1(cfblk1)
  cfblk13/1 -> cfblk14/1

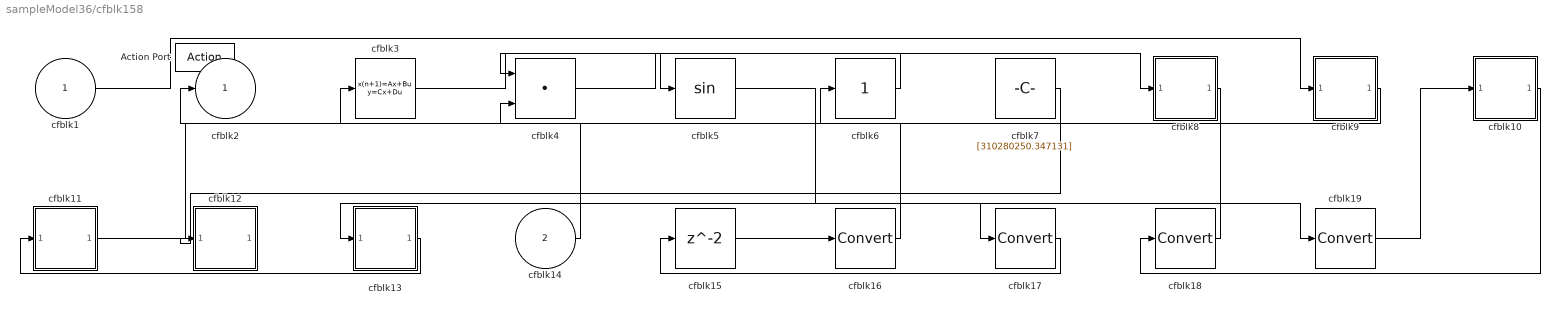
== system sampleModel36/cfblk158 ==
  cfblk1 : Inport
  cfblk14 : Inport  Port=2
  Action Port : ActionPort  ActionType=then
  cfblk10 : Subsystem
  cfblk11 : Subsystem
  cfblk12 : Subsystem
  cfblk13 : Subsystem
  cfblk15 : Delay
  cfblk{16..19} (4 alike) : DataTypeConversion
  cfblk3 : DiscreteStateSpace  SampleTime=-1
  cfblk4 : DotProduct  InputSameDT=on  OutDataTypeStr=Inherit: Inherit via internal rule
  cfblk5 : Trigonometry
  cfblk6 : simulink/Math Operations/Slider Gain  gain=1  low=0  high=2
  cfblk7 : Constant  Value=[310280250.347131]  SampleTime=1
  cfblk8 : Subsystem
  cfblk9 : Subsystem
  cfblk2 : Outport
  wires:
  cfblk11/1(cfblk2) -> cfblk6/1
  cfblk3/1 -> cfblk5/1
  cfblk1/1 -> cfblk9/1(cfblk1)
  cfblk7/1 -> cfblk12/1(cfblk1)
  cfblk4/1 -> cfblk8/1(cfblk1)
  cfblk9/1(cfblk2) -> cfblk2/1
  cfblk6/1 -> cfblk4/1
  cfblk13/1(cfblk2) -> cfblk11/1(cfblk1)
  cfblk14/1 -> cfblk4/2
  cfblk15/1 -> cfblk16/1
  cfblk16/1 -> cfblk3/1
  cfblk8/1(cfblk2) -> cfblk17/1
  cfblk17/1 -> cfblk15/1
  cfblk10/1(cfblk2) -> cfblk18/1
  cfblk18/1 -> cfblk13/1(cfblk1)
  cfblk5/1 -> cfblk19/1
  cfblk19/1 -> cfblk10/1(cfblk1)

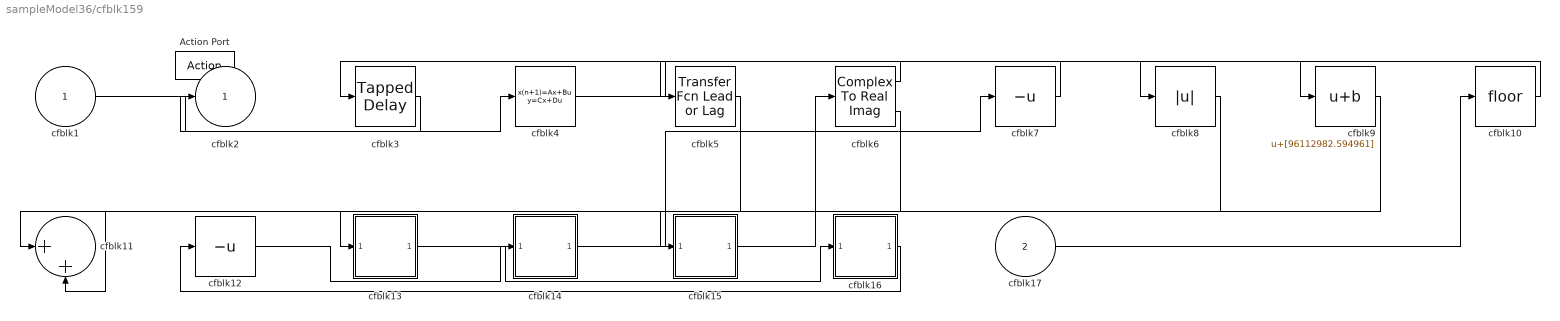
== system sampleModel36/cfblk159 ==
  cfblk1 : Inport
  cfblk17 : Inport  Port=2
  Action Port : ActionPort  ActionType=else
  cfblk10 : Rounding
  cfblk11 : Sum  Inputs=|++
  cfblk12 : UnaryMinus
  cfblk13 : Subsystem
  cfblk14 : Subsystem
  cfblk15 : Subsystem
  cfblk16 : Subsystem
  cfblk3 : simulink/Discrete/Tapped Delay  vinit=0.0  samptime=-1  NumDelays=1  DelayOrder=Oldest  includeCurrent=off
  cfblk4 : DiscreteStateSpace  SampleTime=-1
  cfblk5 : simulink/Discrete/Transfer Fcn Lead or Lag  PoleZ=0.95  ZeroZ=0.75  ICPrevOutput=0.0  ICPrevInput=0.0  DoSatur=off
      settings: SourceProductName=Simulink  SourceProductBaseCode=SL
  cfblk6 : ComplexToRealImag
  cfblk7 : UnaryMinus
  cfblk8 : Abs
  cfblk9 : Bias  Bias=[96112982.594961]
  cfblk2 : Outport
  wires:
  cfblk1/1 -> cfblk4/1
  cfblk10/1 -> cfblk8/1
  cfblk7/1 -> cfblk3/1
  cfblk8/1 -> cfblk13/1(cfblk1)
  cfblk4/1 -> cfblk9/1
  cfblk13/1(cfblk2) -> cfblk16/1(cfblk1)
  cfblk12/1 -> cfblk14/1(cfblk1)
  cfblk16/1(cfblk2) -> cfblk12/1
  cfblk15/1(cfblk2) -> cfblk6/1
  cfblk6/1 -> cfblk5/1
  cfblk14/1(cfblk2) -> cfblk7/1
  cfblk6/2 -> cfblk11/1
  cfblk17/1 -> cfblk10/1
  cfblk9/1 -> cfblk15/1(cfblk1)
  cfblk3/1 -> cfblk2/1
  cfblk5/1 -> cfblk11/2

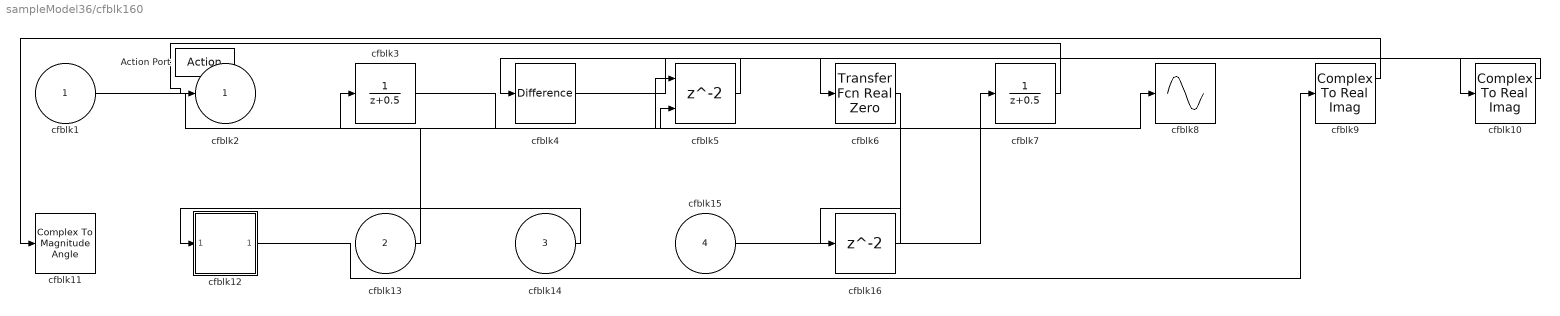
== system sampleModel36/cfblk160 ==
  cfblk1 : Inport
  cfblk13 : Inport  Port=2
  cfblk14 : Inport  Port=3
  cfblk15 : Inport  Port=4
  Action Port : ActionPort  ActionType=then
  cfblk10 : ComplexToRealImag
  cfblk11 : ComplexToMagnitudeAngle
  cfblk12 : Subsystem
  cfblk16 : Delay
  cfblk3 : DiscreteTransferFcn
  cfblk4 : simulink/Discrete/Difference  ICPrevInput=0.0  OutMin=[]  OutMax=[]  OutDataTypeStr=Inherit: Inherit via back propagation  OutDataType=fixdt(1, 16)  OutScaling=2^-10  DoSatur=off
  cfblk5 : Delay  ShowEnablePort=on
      settings: InputPortMap=u0,e6
  cfblk6 : simulink/Discrete/Transfer Fcn Real Zero  ZeroZ=0.75  ICPrevInput=0.0  DoSatur=off
      settings: SourceProductName=Simulink  SourceProductBaseCode=SL
  cfblk7 : DiscreteTransferFcn
  cfblk8 : Sin  TimeSource=Use external signal  SampleTime=0
  cfblk9 : ComplexToRealImag
  cfblk2 : Outport
  wires:
  cfblk5/1 -> cfblk4/1
  cfblk14/1 -> cfblk12/1(cfblk1)
  cfblk1/1 -> cfblk8/1
  cfblk15/1 -> cfblk7/1
  cfblk12/1(cfblk2) -> cfblk9/1
  cfblk7/1 -> cfblk2/1
  cfblk13/1 -> cfblk3/1
  cfblk9/1 -> cfblk11/1
  cfblk10/1 -> cfblk6/1
  cfblk4/1 -> cfblk10/1
  cfblk3/1 -> cfblk5/2
  cfblk6/1 -> cfblk16/1
  cfblk16/1 -> cfblk5/1

== system sampleModel36/cfblk161 ==
  cfblk1 : Inport
  cfblk9 : Inport  Port=2
  Action Port : ActionPort  ActionType=else
  cfblk11 : Subsystem  TreatAsAtomicUnit=on
  cfblk12 : Subsystem  TreatAsAtomicUnit=on
  cfblk3 : DiscreteFir
  cfblk4 : Delay  DelayLengthSource=Input port
      settings: InputPortMap=u0,p1
  cfblk5 : Constant  Value=[947929938.308323]  SampleTime=1
  cfblk6 : Subsystem
  cfblk7 : Subsystem
  cfblk8 : If  IfExpression=u1 >= 0  SampleTime=1
  cfblk2 : Outport
  cfblk10 : Outport  Port=2
  wires:
  cfblk12/1(cfblk2) -> cfblk7/1(cfblk1), cfblk11/2(cfblk8), cfblk11/3(cfblk9)
  cfblk7/1(cfblk2) -> cfblk6/1(cfblk1)
  cfblk1/1 -> cfblk3/1
  cfblk11/1(cfblk2) -> cfblk2/1
  cfblk6/1(cfblk2) -> cfblk10/1
  cfblk4/1 -> cfblk12/1(cfblk1)
  cfblk5/1 -> cfblk11/1(cfblk1)
  cfblk3/1 -> cfblk8/1, cfblk4/2
  cfblk9/1 -> cfblk4/1
  cfblk8/1 -> cfblk11/Action
  cfblk8/2 -> cfblk12/Action

== system sampleModel36/cfblk162 ==
  cfblk1 : Inport
  cfblk8 : Inport  Port=2
  cfblk9 : Inport  Port=3
  Action Port : ActionPort  ActionType=then
  cfblk3 : Constant  Value=[551318933.658010]  SampleTime=1
  cfblk4 : Constant  Value=[-399953801.004817]  SampleTime=1
  cfblk5 : Subsystem
  cfblk6 : Subsystem
  cfblk7 : Subsystem
  cfblk2 : Outport
  wires:
  cfblk1/1 -> cfblk7/1(cfblk1)
  cfblk3/1 -> cfblk6/1(cfblk1)
  cfblk9/1 -> cfblk2/1
  cfblk8/1 -> cfblk5/1(cfblk1)

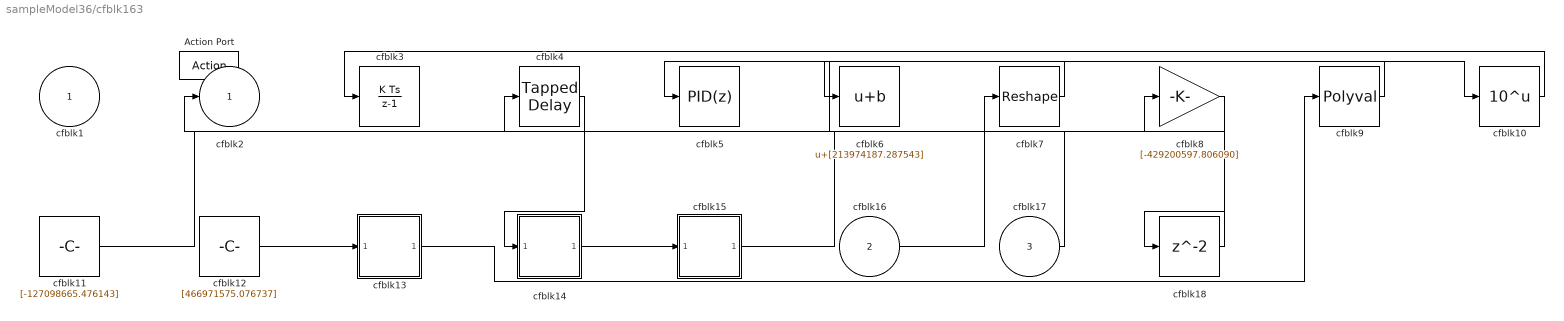
== system sampleModel36/cfblk163 ==
  cfblk1 : Inport
  cfblk16 : Inport  Port=2
  cfblk17 : Inport  Port=3
  Action Port : ActionPort  ActionType=else
  cfblk10 : Math  Operator=10^u  SaturateOnIntegerOverflow=on
  cfblk11 : Constant  Value=[-127098665.476143]  SampleTime=1
  cfblk12 : Constant  Value=[466971575.076737]  SampleTime=1
  cfblk13 : Subsystem
  cfblk14 : Subsystem
  cfblk15 : Subsystem
  cfblk18 : Delay
  cfblk3 : DiscreteIntegrator  SampleTime=-1  ICPrevOutput=DiscIntNeverNeededParam  ICPrevScaledInput=DiscIntNeverNeededParam
  cfblk4 : simulink/Discrete/Tapped Delay  vinit=0.0  samptime=-1  NumDelays=1  DelayOrder=Oldest  includeCurrent=off
  cfblk5 : simulink/Continuous/PID Controller  Controller=PID  TimeDomain=Discrete-time  SampleTime=-1  IntegratorMethod=Forward Euler  FilterMethod=Forward Euler  Form=Parallel  UseFilter=on  ControllerParametersSource=internal  P=1  I=1  D=0  N=100  InitialConditionSource=internal  InitialConditionForIntegrator=0  InitialConditionForFilter=0  ExternalReset=none  LimitOutput=off  UpperSaturationLimit=inf  LowerSaturationLimit=-inf  LinearizeAsGain=off  AntiWindupMode=none  Kb=1  TrackingMode=off  Kt=1  PParamMin=[]  PParamMax=[]  IParamMin=[]  IParamMax=[]  DParamMin=[]  DParamMax=[]  NParamMin=[]  NParamMax=[]  KbParamMin=[]  KbParamMax=[]  KtParamMin=[]  KtParamMax=[]  POutMin=[]  POutMax=[]  IOutMin=[]  IOutMax=[]  DOutMin=[]  DOutMax=[]  NOutMin=[]  NOutMax=[]  KbOutMin=[]  KbOutMax=[]  KtOutMin=[]  KtOutMax=[]  IntegratorOutMin=[]  IntegratorOutMax=[]  FilterOutMin=[]  FilterOutMax=[]  SumOutMin=[]  SumOutMax=[]  SumI1OutMin=[]  SumI1OutMax=[]  SumI2OutMin=[]  SumI2OutMax=[]  SumI3OutMin=[]  SumI3OutMax=[]  SumDOutMin=[]  SumDOutMax=[]  SaturationOutMin=[]  SaturationOutMax=[]  IntegratorContinuousStateAttributes=''  IntegratorStateMustResolveToSignalObject=off  IntegratorRTWStateStorageClass=Auto  FilterContinuousStateAttributes=''  FilterStateMustResolveToSignalObject=off  FilterRTWStateStorageClass=Auto  DifferentiatorICPrevScaledInput=0  DifferentiatorOutMin=[]  DifferentiatorOutMax=[]  FilterDiffOutCoefMin=[]  FilterDiffOutCoefMax=[]  SumDenOutMin=[]  SumDenOutMax=[]  SumNumOutMin=[]  SumNumOutMax=[]  ReciprocalOutMin=[]  ReciprocalOutMax=[]  DivideOutMin=[]  DivideOutMax=[]  TunerSelectOption=Transfer Function Based (PID Tuner App)
  cfblk6 : Bias  Bias=[213974187.287543]
  cfblk7 : Reshape
  cfblk8 : Gain  Gain=[-429200597.806090]
  cfblk9 : Polyval  Coefs=[ +2.081618890e-019, -1.441693666e-014, +4.719686976e-010, -8.536869453e-006, +1.621573104e-001, -8.087801117e+001 ]
  cfblk2 : Outport
  wires:
  cfblk15/1(cfblk2) -> cfblk8/1
  cfblk11/1 -> cfblk10/1
  cfblk7/1 -> cfblk6/1
  cfblk4/1 -> cfblk14/1(cfblk1)
  cfblk9/1 -> cfblk5/1
  cfblk12/1 -> cfblk13/1(cfblk1)
  cfblk10/1 -> cfblk3/1
  cfblk13/1(cfblk2) -> cfblk9/1
  cfblk14/1(cfblk2) -> cfblk15/1(cfblk1)
  cfblk17/1 -> cfblk2/1
  cfblk16/1 -> cfblk7/1
  cfblk8/1 -> cfblk18/1
  cfblk18/1 -> cfblk4/1

== system sampleModel36/cfblk164 ==
  cfblk1 : Inport
  cfblk8 : Inport  Port=2
  cfblk9 : Inport  Port=3
  Action Port : ActionPort  ActionType=then
  cfblk3 : Sin  TimeSource=Use external signal  SampleTime=0
  cfblk4 : Sqrt  Operator=rSqrt  AlgorithmType=Newton-Raphson  SaturateOnIntegerOverflow=on
  cfblk5 : Subsystem
  cfblk6 : Subsystem
  cfblk7 : Subsystem
  cfblk2 : Outport
  wires:
  cfblk8/1 -> cfblk4/1
  cfblk1/1 -> cfblk5/1(cfblk1)
  cfblk9/1 -> cfblk7/1(cfblk1)
  cfblk3/1 -> cfblk2/1
  cfblk5/1(cfblk2) -> cfblk3/1
  cfblk4/1 -> cfblk6/1(cfblk1)

== system sampleModel36/cfblk165 ==
  cfblk1 : Inport
  cfblk8 : Inport  Port=2
  cfblk9 : Inport  Port=3
  cfblk10 : Inport  Port=4
  Action Port : ActionPort  ActionType=else
  cfblk3 : Rounding
  cfblk4 : Sum  Inputs=|++
  cfblk5 : DotProduct  InputSameDT=on  OutDataTypeStr=Inherit: Inherit via internal rule
  cfblk6 : Constant  Value=[955862645.972648]  SampleTime=1
  cfblk7 : Constant  Value=[-868509042.448899]  SampleTime=1
  cfblk2 : Outport
  cfblk11 : Outport  Port=2
  cfblk12 : Outport  Port=3
  cfblk13 : Outport  Port=4
  wires:
  cfblk5/1 -> cfblk4/1
  cfblk1/1 -> cfblk3/1
  cfblk4/1 -> cfblk2/1
  cfblk9/1 -> cfblk12/1
  cfblk8/1 -> cfblk13/1
  cfblk7/1 -> cfblk11/1
  cfblk6/1 -> cfblk5/1
  cfblk10/1 -> cfblk5/2
  cfblk3/1 -> cfblk4/2

== system sampleModel36/cfblk146/cfblk10 ==
  cfblk1 : Inport
  cfblk2 : Outport
  wires:
  cfblk1/1 -> cfblk2/1

== system sampleModel36/cfblk146/cfblk11 ==
  cfblk1 : Inport
  cfblk2 : Outport
  wires:
  cfblk1/1 -> cfblk2/1

== system sampleModel36/cfblk146/cfblk12 ==
  cfblk1 : Inport
  cfblk2 : Outport
  wires:
  cfblk1/1 -> cfblk2/1

== system sampleModel36/cfblk147/cfblk10 ==
  cfblk1 : Inport
  cfblk2 : Outport
  wires:
  cfblk1/1 -> cfblk2/1

== system sampleModel36/cfblk147/cfblk11 ==
  cfblk1 : Inport
  cfblk2 : Outport
  wires:
  cfblk1/1 -> cfblk2/1

== system sampleModel36/cfblk147/cfblk12 ==
  cfblk1 : Inport
  cfblk2 : Outport
  wires:
  cfblk1/1 -> cfblk2/1

== system sampleModel36/cfblk147/cfblk13 ==
  cfblk1 : Inport
  cfblk2 : Outport
  wires:
  cfblk1/1 -> cfblk2/1

== system sampleModel36/cfblk148/cfblk8 ==
  cfblk1 : Inport
  cfblk2 : Outport
  wires:
  cfblk1/1 -> cfblk2/1

== system sampleModel36/cfblk148/cfblk9 ==
  cfblk1 : Inport
  cfblk2 : Outport
  wires:
  cfblk1/1 -> cfblk2/1

== system sampleModel36/cfblk149/cfblk13 ==
  cfblk1 : Inport
  cfblk10 : Inport  Port=2
  cfblk11 : Inport  Port=3
  cfblk12 : Inport  Port=4
  Action Port : ActionPort  ActionType=then
  cfblk3 : Rounding
  cfblk4 : Sum  Inputs=+-
  cfblk5 : Polyval  Coefs=[ +2.081618890e-019, -1.441693666e-014, +4.719686976e-010, -8.536869453e-006, +1.621573104e-001, -8.087801117e+001 ]
  cfblk6 : Subsystem
  cfblk7 : Subsystem
  cfblk8 : Subsystem
  cfblk9 : Subsystem
  cfblk2 : Outport
  cfblk13 : Outport  Port=2
  wires:
  cfblk3/1 -> cfblk13/1
  cfblk5/1 -> cfblk2/1
  cfblk7/1(cfblk2) -> cfblk6/1(cfblk1)
  cfblk11/1 -> cfblk7/1(cfblk1)
  cfblk12/1 -> cfblk3/1
  cfblk1/1 -> cfblk9/1(cfblk1)
  cfblk9/1(cfblk2) -> cfblk8/1(cfblk1)
  cfblk4/1 -> cfblk5/1
  cfblk10/1 -> cfblk4/1
  cfblk6/1(cfblk2) -> cfblk4/2
